simulink model "lab4_simulation"  (R2023a)
settings: Solver=VariableStepAuto  StartTime=0.0  StopTime=10.0  RelTol=1e-3
values from neighbouring files (symbols this model uses):
  den = conv([1, 9], [1, 14])    [lab4.m]
  num = 1.25    [lab4.m]
  P = H21.Numerator    [lab4.m]
  Tm = 3    [lab4.m]
undefined symbols (not defined in the file or in its folder): DENk, NUMk
settings Model: Creator=evely  LastModifiedBy=evely

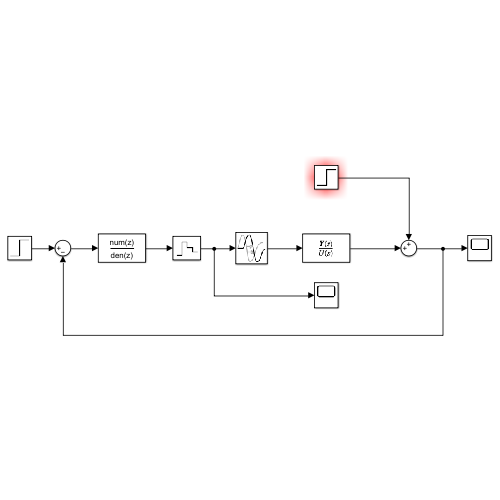
[thumbnail: Simulink's stored preview of the top-level diagram]
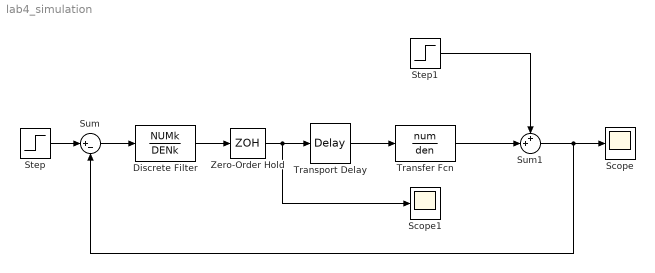
== system lab4_simulation ==
  Discrete Filter : DiscreteFilter  Numerator=NUMk  Denominator=DENk
  Scope : Scope
  Scope1 : Scope
  Step : Step  SampleTime=0
  Step1 : Step  After=P  SampleTime=0
  Sum : Sum  Inputs=|+-
  Sum1 : Sum  Inputs=++|
  Transfer Fcn : TransferFcn  Numerator=num  Denominator=den
  Transport Delay : TransportDelay  DelayTime=Tm
  Zero-Order Hold : ZeroOrderHold  SampleTime=-1
  wires:
  Step/1 -> Sum/1
  Discrete Filter/1 -> Zero-Order Hold/1
  Sum/1 -> Discrete Filter/1
  Zero-Order Hold/1 -> Scope1/1, Transport Delay/1
  Transport Delay/1 -> Transfer Fcn/1
  Sum1/1 -> Sum/2, Scope/1
  Transfer Fcn/1 -> Sum1/2
  Step1/1 -> Sum1/1
